simulink model "Design_of_an_Energy_Efficient_Hybrid_Electric_Vehicle"  (R2023a)
settings: Solver=FixedStepDiscrete  StartTime=0  StopTime=110  RelTol=1e-3  EnableMultiTasking=on
PreLoadFcn:
  | power_motordrive_IPMSM_FOC_data
InitFcn:
  | power_motordrive_IPMSM_FOC_data
  | Cdc  = 0.001;      % DC-link capacitor  [F]
  | AH0  = 280;        % Initial battery charge [hr*A]
  | Tmax=410;
  | 
  | %% Vehicle Parameters for Vehicle Dynamics 2
  | vehicle_mass = 2111;
  | wheel_radius = 0.228;
  | area =2.22;
  | drag_coefficient = 0.23;
  | air_density = 1.204;
  | gravity = 9.81;
  | rolling_res_ratio = 0.02;
  | 
  | % Differential drive parameters
  | gear_ratio = 5;
  | i_t   = gear_ratio ;
  | Rw=wheel_radius;
  | 
  | 
  | %% Sliding Mode Observer
  | pmsm.N_max=wmax;
  | pmsm.p=p
  | pmsm.Ld=Ld;
  | pmsm.Lq=Lq;
  | pmsm.Rs=Rs;
  | PU_System.V_base=(Vdc_nom/sqrt(3));
  | PU_System.I_base=lambda/(Lq-Ld);
  | max_torque=400
  | force_max_pedal=500
  | braking_torque_to_pedal_force_ratio=-4
undefined symbols (not defined in the file): BlkSampleTime, CurrentObserverGain, dataType, DiscIntNeverNeededParam, Fsw, gcbh, Ki_Ireg, Ki_wreg, Kp_Ireg, Kp_wreg, L_smo_gain, lambda, Ld, Limit_Ireg, Limit_wreg, Lq, MaxApplicationSpeed, MaxStatorCurrent, MaxStatorVoltage, NumBits1, NumBits2, p, Pmsm, PolePairs, QPLL, rpm_data, Sensorless, sigbuilder_block, SlidingLimit, Slope1, Slope2, sps_rtmsupport, StatorInductance, StatorResistance, Tmax_data, Tnom, Ts, Vdc_nom, wmax
libraries: fl_lib x27, nesl_utility x24, simulink x23, mcbcontrolslib x15, fl_ps_legacy_lib x9, spsStairGeneratorLib x7, sdl_lib x6, ee_lib x4, mcbpositiondecoderlib x4, BoomBox x3, tiiqmathlib x2, autolibshared x2
(part 4 of 4)

== system Design_of_an_Energy_Efficient_Hybrid_Electric_Vehicle/FOC/Speed Regulator1/Calculate position and speed/Sliding Mode Observer/EEMF Model/angleCompensation ==
  A : Inport
  B : Inport  Port=2
  C : Inport  Port=3
  D : Inport  Port=4
  Bias : Bias  Bias=single(2*pi)  SaturateOnIntegerOverflow=off
  Data Type Duplicate : DataTypeDuplicate  NumInputPorts=6
  Data Type Propagation : simulink/Signal Attributes/Data Type Propagation  PropDataType=fixdt(1, 16)  IfRefDouble=double  IfRefSingle=single  IsSigned=IsSigned1 or IsSigned2  NumBitsBase=max([NumBits1 NumBits2])  NumBitsMult=1  NumBitsAdd=0  NumBitsAllowFinal=1:128  PropScalingMode=Obtain via best precision  PropScaling=2^-10  ValuesUsedBestPrec=[2*pi -2*pi]  SlopeBase=min([Slope1 Slope2])  SlopeMult=1  SlopeAdd=0  BiasBase=Bias1  BiasMult=1  BiasAdd=0
  Data Type Conversion : DataTypeConversion  SaturateOnIntegerOverflow=off  RndMeth=Floor
  Product{,1..3} (4 alike) : Product  OutDataTypeStr=Inherit: Inherit via back propagation
  Scope : Scope
  Sum1 : Sum  Inputs=|++  OutDataTypeStr=Inherit: Same as first input
  Sum2 : Sum  Inputs=|+-  OutDataTypeStr=Inherit: Same as first input
  Switch : Switch  Criteria=u2 > Threshold  SaturateOnIntegerOverflow=off  InputSameDT=off
  atan1 : mcbcontrolslib/atan2  outputUnit=Radians
  Theta : Outport
  wires:
  Data Type Conversion/1 -> Bias/1, Data Type Propagation/3, Switch/2, Switch/1
  Sum1/1 -> atan1/1
  Sum2/1 -> atan1/2
  B/1 -> Product1/1, Product2/1
  atan1/1 -> Scope/1, Data Type Conversion/1, Data Type Propagation/2, Data Type Propagation/1
  D/1 -> Product1/2, Product/2, Data Type Duplicate/6
  C/1 -> Product3/2, Data Type Duplicate/1, Product2/2
  A/1 -> Product3/1, Product/1
  Product2/1 -> Sum1/2, Data Type Duplicate/4
  Switch/1 -> Theta/1
  Bias/1 -> Switch/3
  Product3/1 -> Sum2/2, Data Type Duplicate/2
  Product/1 -> Sum1/1, Data Type Duplicate/5
  Product1/1 -> Sum2/1, Data Type Duplicate/3

== system Design_of_an_Energy_Efficient_Hybrid_Electric_Vehicle/FOC/Speed Regulator1/Calculate position and speed/Sliding Mode Observer/Sliding Mode Observer/Direction_Latch ==
  SigmaAlpha : Inport
  SigmaBeta : Inport  Port=2
  Compare To Zero : simulink/Logic and Bit Operations/Compare To Zero  relop=>  OutDataTypeStr=boolean
  Compare To Zero1 : simulink/Logic and Bit Operations/Compare To Zero  relop=>  OutDataTypeStr=boolean
  Dir_Sense : Subsystem  TreatAsAtomicUnit=on
  If : If
  Merge : Merge
  Merge1 : Merge
  Subsystem2 : Subsystem
  Subsystem3 : Subsystem
  A : Outport
  B : Outport  Port=2
  wires:
  Dir_Sense/1(Sign) -> If/1
  Compare To Zero/1 -> Dir_Sense/1(A), Dir_Sense/Trigger
  Compare To Zero1/1 -> Dir_Sense/2(B)
  Merge/1 -> A/1
  Merge1/1 -> B/1
  Subsystem2/2(Out2) -> Merge1/1
  Subsystem3/1(Out2) -> Merge1/2
  If/2 -> Subsystem3/Action
  Subsystem3/2(Out1) -> Merge/2
  Subsystem2/1(Out1) -> Merge/1
  If/1 -> Subsystem2/Action
  SigmaBeta/1 -> Compare To Zero1/1, Subsystem2/2(SigmaBeta), Subsystem3/1(SigmaBeta)
  SigmaAlpha/1 -> Subsystem3/2(SigmaAlpha), Subsystem2/1(SigmaAlpha), Compare To Zero/1

== system Design_of_an_Energy_Efficient_Hybrid_Electric_Vehicle/FOC/Speed Regulator1/Calculate position and speed/Sliding Mode Observer/Sliding Mode Observer/Subsystem ==
  note: Back Emf computation
  note: Ialpha Estimation
  Valpha : Inport
  Ialpha : Inport  Port=2
  Reset : Inport  Port=3
  Data Type Duplicate : DataTypeDuplicate
  Data Type Duplicate1 : DataTypeDuplicate  NumInputPorts=3
  Data Type Propagation : simulink/Signal Attributes/Data Type Propagation  PropDataType=fixdt(1, 16)  IfRefDouble=double  IfRefSingle=single  IsSigned=IsSigned1 or IsSigned2  NumBitsBase=max([NumBits1 NumBits2])  NumBitsMult=1  NumBitsAdd=0  NumBitsAllowFinal=1:128  PropScalingMode=Obtain via best precision  PropScaling=2^-10  ValuesUsedBestPrec=[SlidingLimit*CurrentObserverGain -SlidingLimit*CurrentObserverGain]  SlopeBase=min([Slope1 Slope2])  SlopeMult=1  SlopeAdd=0  BiasBase=Bias1  BiasMult=1  BiasAdd=0
  Delay : Delay  DelayLength=1  ExternalReset=Level
      settings: InputPortMap=u0,r5
  Delay1 : Delay  DelayLength=1  ExternalReset=Level
      settings: InputPortMap=u0,r5
  Foc_gain : Gain  Gain=single(CurrentObserverGain)  OutDataTypeStr=Inherit: Inherit via back propagation
  Gain : Gain  Gain=single((1/StatorResistance)*(1-exp(-StatorResistance*BlkSampleTime(1)/StatorInductance))*(MaxStatorVoltage/sqrt(3))/MaxStatorCurrent)  OutDataTypeStr=Inherit: Same as input
  Gain1 : Gain  Gain=single(exp(-StatorResistance*BlkSampleTime(1)/StatorInductance))  OutDataTypeStr=Inherit: Same as input
  Gain2 : Gain  Gain=single(2*pi*MaxApplicationSpeed*PolePairs*(1/60)*2*BlkSampleTime(1))  OutDataTypeStr=Inherit: Same as input
  Saturation : Saturate  UpperLimit=SlidingLimit  LowerLimit=-1*SlidingLimit
  Sum : Sum  Inputs=|-+  OutDataTypeStr=Inherit: Same as first input
  Sum1 : Sum  Inputs=+-|  OutDataTypeStr=Inherit: Same as first input
  Sum2 : Sum  OutDataTypeStr=Inherit: Same as first input
  Sum3 : Sum  Inputs=-+|  OutDataTypeStr=Inherit: Same as first input
  Sum4 : Sum  Inputs=++|  OutDataTypeStr=Inherit: Inherit via back propagation
  SigmaAlpha : Outport  VectorParamsAs1DForOutWhenUnconnected=off
  wires:
  Reset/1 -> Delay/2, Delay1/2
  Sum/1 -> Saturation/1, Data Type Propagation/2, Data Type Propagation/1
  Ialpha/1 -> Sum/1, Data Type Duplicate1/1
  Valpha/1 -> Sum1/1, Data Type Duplicate/1
  Gain1/1 -> Sum2/2
  Gain/1 -> Sum2/1, Data Type Duplicate1/3
  Sum1/1 -> Gain/1
  Delay/1 -> Gain1/1
  Sum4/1 -> Delay1/1, Data Type Duplicate/2
  Sum2/1 -> Delay/1, Sum/2, Data Type Duplicate1/2
  Delay1/1 -> Sum1/2, Sum3/1, SigmaAlpha/1, Sum4/1
  Saturation/1 -> Foc_gain/1
  Foc_gain/1 -> Data Type Propagation/3, Sum3/2
  Sum3/1 -> Gain2/1
  Gain2/1 -> Sum4/2

== system Design_of_an_Energy_Efficient_Hybrid_Electric_Vehicle/FOC/Speed Regulator1/Calculate position and speed/Sliding Mode Observer/Sliding Mode Observer/Subsystem1 ==
  note: Back Emf computation
  note: Ibeta Estimation
  Vbeta : Inport
  Ibetaa : Inport  Port=2
  Reset : Inport  Port=3
  Data Type Duplicate : DataTypeDuplicate
  Data Type Duplicate1 : DataTypeDuplicate  NumInputPorts=3
  Data Type Propagation : simulink/Signal Attributes/Data Type Propagation  PropDataType=fixdt(1, 16)  IfRefDouble=double  IfRefSingle=single  IsSigned=IsSigned1 or IsSigned2  NumBitsBase=max([NumBits1 NumBits2])  NumBitsMult=1  NumBitsAdd=0  NumBitsAllowFinal=1:128  PropScalingMode=Obtain via best precision  PropScaling=2^-10  ValuesUsedBestPrec=[SlidingLimit*CurrentObserverGain -SlidingLimit*CurrentObserverGain]  SlopeBase=min([Slope1 Slope2])  SlopeMult=1  SlopeAdd=0  BiasBase=Bias1  BiasMult=1  BiasAdd=0
  Delay : Delay  DelayLength=1  ExternalReset=Level
      settings: InputPortMap=u0,r5
  Delay1 : Delay  DelayLength=1  ExternalReset=Level
      settings: InputPortMap=u0,r5
  Foc_gain : Gain  Gain=single(CurrentObserverGain)  OutDataTypeStr=Inherit: Inherit via back propagation
  Gain : Gain  Gain=single((1/StatorResistance)*(1-exp(-StatorResistance*BlkSampleTime(1)/StatorInductance))*(MaxStatorVoltage/sqrt(3))/MaxStatorCurrent)  OutDataTypeStr=Inherit: Same as input
  Gain1 : Gain  Gain=single(exp(-StatorResistance*BlkSampleTime(1)/StatorInductance))  OutDataTypeStr=Inherit: Same as input
  Gain2 : Gain  Gain=single(2*pi*MaxApplicationSpeed*PolePairs*(1/60)*2*BlkSampleTime(1))  OutDataTypeStr=Inherit: Same as input
  Saturation : Saturate  UpperLimit=SlidingLimit  LowerLimit=-1*SlidingLimit
  Sum : Sum  Inputs=|-+  OutDataTypeStr=Inherit: Same as first input
  Sum1 : Sum  Inputs=+-|  OutDataTypeStr=Inherit: Same as first input
  Sum2 : Sum  OutDataTypeStr=Inherit: Same as first input
  Sum3 : Sum  Inputs=-+|  OutDataTypeStr=Inherit: Same as first input
  Sum4 : Sum  Inputs=++|  OutDataTypeStr=Inherit: Inherit via back propagation
  SigmaBeta : Outport  VectorParamsAs1DForOutWhenUnconnected=off
  wires:
  Reset/1 -> Delay1/2, Delay/2
  Sum/1 -> Saturation/1, Data Type Propagation/2, Data Type Propagation/1
  Ibetaa/1 -> Sum/1, Data Type Duplicate1/1
  Vbeta/1 -> Sum1/1, Data Type Duplicate/1
  Gain1/1 -> Sum2/2
  Saturation/1 -> Foc_gain/1
  Gain/1 -> Sum2/1, Data Type Duplicate1/3
  Sum1/1 -> Gain/1
  Foc_gain/1 -> Sum3/2, Data Type Propagation/3
  Delay/1 -> Gain1/1
  Sum4/1 -> Delay1/1, Data Type Duplicate/2
  Sum2/1 -> Delay/1, Sum/2, Data Type Duplicate1/2
  Delay1/1 -> Sum1/2, Sum3/1, SigmaBeta/1, Sum4/1
  Sum3/1 -> Gain2/1
  Gain2/1 -> Sum4/2

== system Design_of_an_Energy_Efficient_Hybrid_Electric_Vehicle/FOC/Speed Regulator1/Calculate position and speed/Sliding Mode Observer/Sliding Mode Observer/angleCompensation ==
  A : Inport
  B : Inport  Port=2
  C : Inport  Port=3
  D : Inport  Port=4
  Bias : Bias  Bias=single(2*pi)  SaturateOnIntegerOverflow=off
  Data Type Duplicate : DataTypeDuplicate  NumInputPorts=6
  Data Type Propagation : simulink/Signal Attributes/Data Type Propagation  PropDataType=fixdt(1, 16)  IfRefDouble=double  IfRefSingle=single  IsSigned=IsSigned1 or IsSigned2  NumBitsBase=max([NumBits1 NumBits2])  NumBitsMult=1  NumBitsAdd=0  NumBitsAllowFinal=1:128  PropScalingMode=Obtain via best precision  PropScaling=2^-10  ValuesUsedBestPrec=[2*pi -2*pi]  SlopeBase=min([Slope1 Slope2])  SlopeMult=1  SlopeAdd=0  BiasBase=Bias1  BiasMult=1  BiasAdd=0
  Data Type Conversion : DataTypeConversion  SaturateOnIntegerOverflow=off  RndMeth=Floor
  Product{,1..3} (4 alike) : Product  OutDataTypeStr=Inherit: Inherit via back propagation
  Sum1 : Sum  Inputs=|++  OutDataTypeStr=Inherit: Same as first input
  Sum2 : Sum  Inputs=|+-  OutDataTypeStr=Inherit: Same as first input
  Switch : Switch  Criteria=u2 > Threshold  SaturateOnIntegerOverflow=off  InputSameDT=off
  atan1 : mcbcontrolslib/atan2  outputUnit=Radians
  Theta : Outport
  wires:
  Data Type Conversion/1 -> Bias/1, Data Type Propagation/3, Switch/2, Switch/1
  Sum1/1 -> atan1/1
  Sum2/1 -> atan1/2
  B/1 -> Product1/1, Product2/1
  atan1/1 -> Data Type Conversion/1, Data Type Propagation/2, Data Type Propagation/1
  D/1 -> Product1/2, Product/2, Data Type Duplicate/6
  C/1 -> Product3/2, Data Type Duplicate/1, Product2/2
  A/1 -> Product3/1, Product/1
  Product2/1 -> Sum1/2, Data Type Duplicate/4
  Switch/1 -> Theta/1
  Bias/1 -> Switch/3
  Product3/1 -> Sum2/2, Data Type Duplicate/2
  Product/1 -> Sum1/1, Data Type Duplicate/5
  Product1/1 -> Sum2/1, Data Type Duplicate/3

== system Design_of_an_Energy_Efficient_Hybrid_Electric_Vehicle/FOC/Speed Regulator1/Calculate position and speed/Sliding Mode Observer/Subsystem/Alpha_loop_current_est ==
  Valpha : Inport
  Ialpha : Inport  Port=2
  Reset1 : Inport  Port=3
  Add : Sum  Inputs=-+
  Eq12_alpha_loop : Subsystem
  Gain3 : Gain  Gain=L_smo_gain  OutDataTypeStr=Inherit: Same as input
  Saturation : Saturate  UpperLimit=SlidingLimit  LowerLimit=-1*SlidingLimit  OutDataTypeStr=single
  Zalpha[k+1] : Outport  VectorParamsAs1DForOutWhenUnconnected=off
  wires:
  Valpha/1 -> Eq12_alpha_loop/2(Valpha*)
  Eq12_alpha_loop/1(Ialpha_est) -> Add/2
  Ialpha/1 -> Add/1
  Add/1 -> Saturation/1
  Saturation/1 -> Gain3/1, Zalpha[k+1]/1
  Gain3/1 -> Eq12_alpha_loop/1(L*Zalpha[k+1])
  Reset1/1 -> Eq12_alpha_loop/3(Reset)

== system Design_of_an_Energy_Efficient_Hybrid_Electric_Vehicle/FOC/Speed Regulator1/Calculate position and speed/Sliding Mode Observer/Subsystem/Beta_loop_current_est ==
  Vbeta : Inport
  Ibeta : Inport  Port=2
  Reset1 : Inport  Port=3
  Add : Sum  Inputs=-+
  Eq12_beta_loop : Subsystem
  Gain3 : Gain  Gain=L_smo_gain  OutDataTypeStr=Inherit: Same as input
  Saturation : Saturate  UpperLimit=SlidingLimit  LowerLimit=-1*SlidingLimit  OutDataTypeStr=single
  Zbeta[k+1] : Outport  VectorParamsAs1DForOutWhenUnconnected=off
  wires:
  Vbeta/1 -> Eq12_beta_loop/2(Vbeta*)
  Eq12_beta_loop/1(Ibeta_est) -> Add/2
  Ibeta/1 -> Add/1
  Add/1 -> Saturation/1
  Saturation/1 -> Gain3/1, Zbeta[k+1]/1
  Gain3/1 -> Eq12_beta_loop/1(L*Zbeta[k+1])
  Reset1/1 -> Eq12_beta_loop/3(Reset)

== system Design_of_an_Energy_Efficient_Hybrid_Electric_Vehicle/FOC/Speed Regulator1/Calculate position and speed/Sliding Mode Observer/Subsystem/QPLL ==
  Zalpha[k+1] : Inport
  Zbeta[k+1] : Inport  Port=2
  Add : Sum
  Add1 : Sum  Inputs=--
  Demux : Demux  Outputs=2
  Divide : Product  Inputs=/*  OutDataTypeStr=double
  Gain2 : Gain  Gain=single(60/((2*pi)*pmsm.N_base*pmsm.p))
  IIR Filter2 : mcbcontrolslib/IIR Filter  VariantControl=Low Pass Filter  VariantSelect=Low-pass  Filter_constant=single(Ts*pmsm.N_max*pmsm.p/120)  advancedSettings=off  Ts=50e-6  cutOff_freq=1
  Math Function : Math  Operator=square
  Math Function1 : Math  Operator=square
  Mux : Mux  Inputs=2
  PI Controller : slpidlib/PID Controller  Controller=PI  Form=Parallel  TimeDomain=Discrete-time  UseExternalTs=off  SampleTime=-1  IntegratorMethod=Forward Euler  FilterMethod=Forward Euler  ControllerParametersSource=internal  P=90  I=300  D=0  UseFilter=on  N=100  TunerSelectOption=Transfer Function Based (PID Tuner App)  InitialConditionSource=internal  InitialConditionForIntegrator=0  InitialConditionForFilter=0  DifferentiatorICPrevScaledInput=0  ExternalReset=none  TrackingMode=off  Kt=1  LimitOutput=off  SatLimitsSource=internal  UpperSaturationLimit=inf  LowerSaturationLimit=0  LinearizeAsGain=off  AntiWindupMode=none  Kb=1  POutMin=[]  POutMax=[]  IOutMin=[]  IOutMax=[]  DOutMin=[]  DOutMax=[]  NOutMin=[]  NOutMax=[]  SumOutMin=[]  SumOutMax=[]  SaturationOutMin=[]  SaturationOutMax=[]  PParamMin=[]  PParamMax=[]  IParamMin=[]  IParamMax=[]  DParamMin=[]  DParamMax=[]  NParamMin=[]  NParamMax=[]  KbParamMin=[]  KbParamMax=[]  KtParamMin=[]  KtParamMax=[]  KbOutMin=[]  KbOutMax=[]  KtOutMin=[]  KtOutMax=[]  IntegratorOutMin=[]  IntegratorOutMax=[]  FilterOutMin=[]  FilterOutMax=[]  SumI1OutMin=[]  SumI1OutMax=[]  SumI2OutMin=[]  SumI2OutMax=[]  SumI3OutMin=[]  SumI3OutMax=[]  SumI4OutMin=[]  SumI4OutMax=[]  SumDOutMin=[]  SumDOutMax=[]  DifferentiatorOutMin=[]  DifferentiatorOutMax=[]  FilterDiffOutCoefMin=[]  FilterDiffOutCoefMax=[]  ReciprocalOutMin=[]  ReciprocalOutMax=[]  SumDenOutMin=[]  SumDenOutMax=[]  SumNumOutMin=[]  SumNumOutMax=[]  DivideOutMin=[]  DivideOutMax=[]  UdiffTsProdOutMin=[]  UdiffTsProdOutMax=[]  NTsProdOutMin=[]  NTsProdOutMax=[]  UintegralTsProdOutMin=[]  UintegralTsProdOutMax=[]  UngainTsProdOutMin=[]  UngainTsProdOutMax=[]  IntegratorContinuousStateAttributes=''  IntegratorStateMustResolveToSignalObject=off  IntegratorRTWStateStorageClass=Auto  FilterContinuousStateAttributes=''  FilterStateMustResolveToSignalObject=off  FilterRTWStateStorageClass=Auto  ParallelPVariant=InternalParameters  IdealPVariant=Disabled  IVariant=InternalParameters  DVariant=Disabled  IntegratorVariant=Discrete  SatVariant=Disabled  AWVariant=Passthrough  PCopyVariant=Disabled  TRVariant=Disabled  FdbkBlocksVariant=Forward  IdealPFdbkVariant=Disabled  SatFdbkVariant=Disabled  DerivativeFilterVariant=Disabled  NVariant=Disabled  NCopyVariant=Disabled_SignalSpec  FilterICVariant=Disabled  IntegratorICVariant=InternalICs  ExternalResetVariant=Disabled  TRSumVariant=Passthrough  SumFdbkVariant=Disabled  SumVariant=Sum_PI  TsampFilterVariant=InternalTs  TsampNgainVariant=Passthrough  TsampIntegralVariant=Passthrough  ExternalSaturationOutDataTypeStr=Inherit: Same as second input
  Product : Product  OutDataTypeStr=Inherit: Inherit via back propagation
  Product1 : Product  OutDataTypeStr=Inherit: Inherit via back propagation
  Scope{1..3,5,7} (5 alike) : Scope  NumInputPorts=2
  Sqrt : Sqrt
  Trigonometric Function : Trigonometry  Operator=cos  OutputSignalType=real
  Trigonometric Function1 : Trigonometry  OutputSignalType=real
  Wrap state discrete Integrator : Subsystem  AncestorBlock=|
      | eeAsmScalarControl/Induction Machine
      | Scalar Control/Wrap state
      | discrete Integrator
      settings: LibrarySourceBlock=|
      | eeAsmScalarControl/Induction Machine
      | Scalar Control/Wrap state
      | discrete Integrator
  y : Outport
  wires:
  Math Function/1 -> Add/1
  Math Function1/1 -> Add/2
  Add/1 -> Sqrt/1
  Demux/1 -> Math Function/1, Product/2, Scope2/1
  Demux/2 -> Math Function1/1, Product1/1, Scope2/2
  Product/1 -> Add1/1
  Product1/1 -> Add1/2
  Divide/1 -> Scope7/2, PI Controller/1
  Zalpha[k+1]/1 -> Mux/2
  Zbeta[k+1]/1 -> Mux/1
  Sqrt/1 -> Divide/1, Scope3/1
  Add1/1 -> Divide/2, Scope7/1
  Trigonometric Function/1 -> Product1/2
  Trigonometric Function1/1 -> Product/1
  Wrap state discrete Integrator/1(y) -> Trigonometric Function/1, Trigonometric Function1/1, Scope1/1, y/1
  Gain2/1 -> Scope1/2
  Mux/1 -> Demux/1
  PI Controller/1 -> IIR Filter2/1, Wrap state discrete Integrator/1(u)
  IIR Filter2/1 -> Gain2/1

== system Design_of_an_Energy_Efficient_Hybrid_Electric_Vehicle/FOC/Speed Regulator1/Calculate position and speed/Sliding Mode Observer (SMO)/Debounce/Speed IIR filter ==
  Speed : Inport
  Add : Sum  Inputs=+-
  Add1 : Sum
  Constant1 : Constant  OutDataTypeStr=fixdt(1,32,17)
  Constant2 : Constant  Value=.01  OutDataTypeStr=fixdt(1,32,17)
  Product : Product  OutDataTypeStr=Inherit: Same as first input
  Product1 : Product  OutDataTypeStr=Inherit: Same as first input
  Unit Delay : UnitDelay  SampleTime=-1  HasFrameUpgradeWarning=on
  Filtered speed : Outport  VectorParamsAs1DForOutWhenUnconnected=off
  wires:
  Speed/1 -> Product/1
  Add1/1 -> Unit Delay/1, Filtered speed/1
  Constant1/1 -> Add/1
  Constant2/1 -> Product/2, Add/2
  Product/1 -> Add1/1
  Add/1 -> Product1/1
  Unit Delay/1 -> Product1/2
  Product1/1 -> Add1/2

== system Design_of_an_Energy_Efficient_Hybrid_Electric_Vehicle/FOC/Speed Regulator1/Calculate position and speed/Sliding Mode Observer/EEMF Model/Direction_Latch/Dir_Sense ==
  A : Inport
  B : Inport  Port=2
  Trigger : TriggerPort  VariantControl=Variant
  Constant : Constant  Value=-1
  Constant1 : Constant
  Logical Operator : Logic  AllPortsSameDT=off  OutDataTypeStr=boolean
  Switch : Switch  Criteria=u2 ~= 0  OutDataTypeStr=int16  SaturateOnIntegerOverflow=off  InputSameDT=off
  Sign : Outport  InitialOutput=0  VectorParamsAs1DForOutWhenUnconnected=off
  wires:
  Switch/1 -> Sign/1
  Constant1/1 -> Switch/3
  Constant/1 -> Switch/1
  Logical Operator/1 -> Switch/2
  B/1 -> Logical Operator/2
  A/1 -> Logical Operator/1

== system Design_of_an_Energy_Efficient_Hybrid_Electric_Vehicle/FOC/Speed Regulator1/Calculate position and speed/Sliding Mode Observer/EEMF Model/Direction_Latch/Subsystem2 ==
  SigmaAlpha : Inport
  SigmaBeta : Inport  Port=2
  Action Port : ActionPort  ActionPortLabel=if(u1 > 0)
  Unary Minus : UnaryMinus
  Out1 : Outport
  Out2 : Outport  Port=2
  wires:
  Unary Minus/1 -> Out1/1
  SigmaBeta/1 -> Out2/1
  SigmaAlpha/1 -> Unary Minus/1

== system Design_of_an_Energy_Efficient_Hybrid_Electric_Vehicle/FOC/Speed Regulator1/Calculate position and speed/Sliding Mode Observer/EEMF Model/Direction_Latch/Subsystem3 ==
  SigmaBeta : Inport
  SigmaAlpha : Inport  Port=2
  Action Port : ActionPort  ActionPortLabel=else
  Unary Minus : UnaryMinus
  Out2 : Outport
  Out1 : Outport  Port=2
  wires:
  Unary Minus/1 -> Out2/1
  SigmaAlpha/1 -> Out1/1
  SigmaBeta/1 -> Unary Minus/1

== system Design_of_an_Energy_Efficient_Hybrid_Electric_Vehicle/FOC/Speed Regulator1/Calculate position and speed/Sliding Mode Observer/EEMF Model/Sliding Mode Observer/2nd order LPF ==
  In : Inport
  reset : Inport  Port=2
  Compute filter constant : Subsystem
  LPF1 : Subsystem  mask(Basic IIR LPF filter){}
      mask help:
      | The output is computed as:
      | y[k] = G * y[k-1] + (1-G) * u[k]
  LPF2 : Subsystem  mask(Basic IIR LPF filter){}
      mask help:
      | The output is computed as:
      | y[k] = G * y[k-1] + (1-G) * u[k]
  Out : Outport
  wires:
  reset/1 -> LPF2/2(rst), LPF1/2(rst)
  In/1 -> LPF1/1(In)
  Compute filter constant/1(G) -> LPF1/3(G), LPF2/3(G)
  LPF1/1(Out) -> LPF2/1(In)
  LPF2/1(Out) -> Out/1

== system Design_of_an_Energy_Efficient_Hybrid_Electric_Vehicle/FOC/Speed Regulator1/Calculate position and speed/Sliding Mode Observer/EEMF Model/Sliding Mode Observer/Back EMF estimation (SMO) ==
  Is_αβ : Inport
  Vs_αβ : Inport  Port=2
  Delay : Delay  DelayLength=1  InitialCondition=0
  Gain1 : Gain  Gain=Rs/Ls
  Gain2 : Gain  Gain=1/Ls
  Gain3 : Gain  Gain=Ks
  Gain4 : Gain  Gain=1/Ls
  Sigmoid : Subsystem
      mask Display: plot(linspace(-1,1,100),(2./(1+exp(-10*linspace(-1,1,100))))-1)
  Sum : Sum  Inputs=|++
  Sum1 : Sum  Inputs=|+-
  Sum2 : Sum  Inputs=|+-
  Sum3 : Sum  Inputs=|-+
  Weighted sample time : SampleTimeMath  TsampMathOp=*  weightValue=1
  Weighted sample time1 : SampleTimeMath  TsampMathOp=*  weightValue=1
  Weighted sample time2 : SampleTimeMath  TsampMathOp=*  weightValue=1
  e_αβ : Outport
  wires:
  Sum/1 -> Sum1/1
  Sum1/1 -> Delay/1
  Sum3/1 -> Sum/1
  Gain4/1 -> Sum/2
  Is_αβ/1 -> Sum2/2
  Vs_αβ/1 -> Weighted sample time1/1
  Delay/1 -> Weighted sample time2/1, Sum3/2, Sum2/1
  Gain3/1 -> e_αβ/1, Weighted sample time/1
  Sum2/1 -> Sigmoid/1(u)
  Sigmoid/1(y) -> Gain3/1
  Weighted sample time/1 -> Gain2/1
  Gain2/1 -> Sum1/2
  Weighted sample time1/1 -> Gain4/1
  Weighted sample time2/1 -> Gain1/1
  Gain1/1 -> Sum3/1

== system Design_of_an_Energy_Efficient_Hybrid_Electric_Vehicle/FOC/Speed Regulator1/Calculate position and speed/Sliding Mode Observer/EEMF Model/Sliding Mode Observer/Speed//position estimation Arctan method ==
  e_αβ : Inport
  reset : Inport  Port=2
  Atan : Trigonometry  Operator=atan2
  Demux : Demux  Outputs=2
  Gain : Gain  Gain=-1
  Rotor mechanical speed : Subsystem  mask{fc=1e3}
      mask prompts: fc "Filter cutoff frequency [Hz]"
      mask help:
      | The rotor speed is obtained by differentiation of the measured angle. The "function block" removes angle discontinuities.
      |
      | The derivative is then filtered to reduce the noise introduced by the numerical differentiation.
      |
      | Additional details can be found in "PN104: Using the angle decoder modules" on the imperix knowledge base (kb.imperix.com).
  Scope1 : Scope
  Scope2 : Scope
  Scope3 : Scope
  ωs : Outport
  θs : Outport  Port=2
  wires:
  Demux/1 -> Atan/1
  Demux/2 -> Atan/2
  e_αβ/1 -> Demux/1
  Atan/1 -> Scope2/1, Gain/1
  Gain/1 -> Rotor mechanical speed/1(angle), θs/1
  Rotor mechanical speed/1(speed) -> Scope3/1, ωs/1
  reset/1 -> Scope1/1, Rotor mechanical speed/2(reset)

== system Design_of_an_Energy_Efficient_Hybrid_Electric_Vehicle/FOC/Speed Regulator1/Calculate position and speed/Sliding Mode Observer/EEMF Model/Sliding Mode Observer/Speed//position estimation Q-PLL method ==
  V_αβ : Inport
  ωc : Inport  Port=2
  Kp : Inport  Port=3
  Ki : Inport  Port=4
  reset : Inport  Port=5
  Constant : Constant  Value=[0 0]  OutDataTypeStr=single
  Demux : Demux  Outputs=2
  PI : Subsystem
  Product : Product
  Product1 : Product
  Sum : Sum  Inputs=|++
  Sum1 : Sum  Inputs=-|+
  Switch : Switch  Criteria=u2 > Threshold  SaturateOnIntegerOverflow=off  InputSameDT=off
  Trigonometric Function : Trigonometry  OutputSignalType=real
  Trigonometric Function1 : Trigonometry  Operator=cos  OutputSignalType=real
  Wrapping integrator : Subsystem
      mask help: The integrator uses the Forward Euler method and wraps its state between 0 and 2*pi.
  ωs : Outport
  θs : Outport  Port=2
  wires:
  reset/1 -> PI/4(Reset), Switch/2
  PI/1(u) -> Sum/1
  Switch/1 -> Demux/1
  V_αβ/1 -> Switch/3
  Constant/1 -> Switch/1
  Trigonometric Function/1 -> Product1/1
  Trigonometric Function1/1 -> Product/2
  Sum1/1 -> PI/1(e)
  Demux/1 -> Product1/2
  Demux/2 -> Product/1
  Wrapping integrator/1(out) -> θs/1, Trigonometric Function1/1, Trigonometric Function/1
  Sum/1 -> Wrapping integrator/1(in), ωs/1
  ωc/1 -> Sum/2
  Kp/1 -> PI/2(Kp)
  Ki/1 -> PI/3(Ki)
  Product1/1 -> Sum1/1
  Product/1 -> Sum1/2

== system Design_of_an_Energy_Efficient_Hybrid_Electric_Vehicle/FOC/Speed Regulator1/Calculate position and speed/Sliding Mode Observer/EEMF Model/Sliding Mode Observer/compensate LPF phase 1 ==
  ωs : Inport
  θ_in : Inport  Port=2
  Add : Sum
  Atan : Trigonometry  Operator=atan2
  Constant1 : Constant  Value=2*pi*fc  OutDataTypeStr=single
  Filter order : Gain  Gain=2
  θ_out : Outport
  wires:
  Constant1/1 -> Atan/2
  ωs/1 -> Atan/1
  Add/1 -> θ_out/1
  Atan/1 -> Filter order/1
  θ_in/1 -> Add/1
  Filter order/1 -> Add/2

== system Design_of_an_Energy_Efficient_Hybrid_Electric_Vehicle/FOC/Speed Regulator1/Calculate position and speed/Sliding Mode Observer/EEMF Model/Sliding Mode Observer/compensate LPF phase 2 ==
  ωs : Inport
  θ_in : Inport  Port=2
  Add : Sum
  Atan : Trigonometry  Operator=atan2
  Constant1 : Constant  Value=2*pi*fc  OutDataTypeStr=single
  Filter order : Gain  Gain=2
  θ_out : Outport
  wires:
  Filter order/1 -> Add/2
  θ_in/1 -> Add/1
  Atan/1 -> Filter order/1
  Add/1 -> θ_out/1
  ωs/1 -> Atan/1
  Constant1/1 -> Atan/2

== system Design_of_an_Energy_Efficient_Hybrid_Electric_Vehicle/FOC/Speed Regulator1/Calculate position and speed/Sliding Mode Observer/EEMF Model/Sliding Mode Observer/compensate PLL phase ==
  θ_in : Inport
  ωc : Inport  Port=2
  Gain : Gain  Gain=pi/2
  Sign : Signum
  Sum : Sum  Inputs=|+-
  θ_out : Outport
  wires:
  θ_in/1 -> Sum/1
  Sum/1 -> θ_out/1
  Sign/1 -> Gain/1
  ωc/1 -> Sign/1
  Gain/1 -> Sum/2

== system Design_of_an_Energy_Efficient_Hybrid_Electric_Vehicle/FOC/Speed Regulator1/Calculate position and speed/Sliding Mode Observer/EEMF Model/Subsystem/shi_1 ==
  In1 : Inport
  Gain : Gain  Gain=-1
  Gain8 : Gain  Gain=single((pmsm.Ld-pmsm.Lq))
  Gain9 : Gain
  Shi1 : Gain  Gain=single((1/pmsm.Rs)*(1-exp(-pmsm.Rs*Ts/pmsm.Ld))*(PU_System.V_base/sqrt(3))/PU_System.I_base)  OutDataTypeStr=Inherit: Same as input
  Out1 : Outport
  wires:
  Gain8/1 -> Out1/1
  Gain9/1 -> Shi1/1
  In1/1 -> Gain/1
  Gain/1 -> Gain9/1
  Shi1/1 -> Gain8/1

== system Design_of_an_Energy_Efficient_Hybrid_Electric_Vehicle/FOC/Speed Regulator1/Calculate position and speed/Sliding Mode Observer/EEMF Model/Subsystem1/shi_1 ==
  In1 : Inport
  Gain : Gain
  Gain8 : Gain  Gain=single((pmsm.Ld-pmsm.Lq))
  Gain9 : Gain
  Shi : Gain  Gain=single((1/pmsm.Rs)*(1-exp(-pmsm.Rs*Ts/pmsm.Ld))*(PU_System.V_base/sqrt(3))/PU_System.I_base)  OutDataTypeStr=Inherit: Same as input
  Out1 : Outport
  wires:
  Gain8/1 -> Out1/1
  Gain9/1 -> Shi/1
  In1/1 -> Gain/1
  Gain/1 -> Gain9/1
  Shi/1 -> Gain8/1

== system Design_of_an_Energy_Efficient_Hybrid_Electric_Vehicle/FOC/Speed Regulator1/Calculate position and speed/Sliding Mode Observer/Sliding Mode Observer/Direction_Latch/Dir_Sense ==
  A : Inport
  B : Inport  Port=2
  Trigger : TriggerPort  VariantControl=Variant
  Constant : Constant  Value=-1
  Constant1 : Constant
  Logical Operator : Logic  AllPortsSameDT=off  OutDataTypeStr=boolean
  Switch : Switch  Criteria=u2 ~= 0  OutDataTypeStr=int16  SaturateOnIntegerOverflow=off  InputSameDT=off
  Sign : Outport  InitialOutput=0  VectorParamsAs1DForOutWhenUnconnected=off
  wires:
  Switch/1 -> Sign/1
  Constant1/1 -> Switch/3
  Constant/1 -> Switch/1
  Logical Operator/1 -> Switch/2
  B/1 -> Logical Operator/2
  A/1 -> Logical Operator/1

== system Design_of_an_Energy_Efficient_Hybrid_Electric_Vehicle/FOC/Speed Regulator1/Calculate position and speed/Sliding Mode Observer/Sliding Mode Observer/Direction_Latch/Subsystem2 ==
  SigmaAlpha : Inport
  SigmaBeta : Inport  Port=2
  Action Port : ActionPort
  Unary Minus : UnaryMinus
  Out1 : Outport
  Out2 : Outport  Port=2
  wires:
  Unary Minus/1 -> Out1/1
  SigmaBeta/1 -> Out2/1
  SigmaAlpha/1 -> Unary Minus/1

== system Design_of_an_Energy_Efficient_Hybrid_Electric_Vehicle/FOC/Speed Regulator1/Calculate position and speed/Sliding Mode Observer/Sliding Mode Observer/Direction_Latch/Subsystem3 ==
  SigmaBeta : Inport
  SigmaAlpha : Inport  Port=2
  Action Port : ActionPort
  Unary Minus : UnaryMinus
  Out2 : Outport
  Out1 : Outport  Port=2
  wires:
  Unary Minus/1 -> Out2/1
  SigmaAlpha/1 -> Out1/1
  SigmaBeta/1 -> Unary Minus/1

== system Design_of_an_Energy_Efficient_Hybrid_Electric_Vehicle/FOC/Speed Regulator1/Calculate position and speed/Sliding Mode Observer/Subsystem/Alpha_loop_current_est/Eq12_alpha_loop ==
  L*Zalpha[k+1] : Inport
  Valpha* : Inport  Port=2
  Reset : Inport  Port=3
  Add1 : Sum
  Add2 : Sum
  Delay1 : Delay  DelayLength=1  ExternalReset=Level
      settings: InputPortMap=u0,r5
  Delay2 : Delay  DelayLength=1  ExternalReset=Level
      settings: InputPortMap=u0,r5
  Gain : Gain  Gain=1/pmsm.Lq
  Gain1 : Gain  Gain=Ts
  Gain2 : Gain  Gain=(1-(Ts*pmsm.Rs/pmsm.Lq))
  Ialpha_est : Outport  VectorParamsAs1DForOutWhenUnconnected=off
  wires:
  Valpha*/1 -> Gain/1
  L*Zalpha[k+1]/1 -> Delay2/1
  Reset/1 -> Delay1/2, Delay2/2
  Delay2/1 -> Add1/1  "L*Zaplha[k]"
  Gain/1 -> Add1/2  "Valpha*/Lq"
  Add1/1 -> Gain1/1
  Delay1/1 -> Gain2/1
  Gain1/1 -> Add2/2
  Gain2/1 -> Add2/1
  Add2/1 -> Ialpha_est/1, Delay1/1  "Ialpha_est[k+1]"

== system Design_of_an_Energy_Efficient_Hybrid_Electric_Vehicle/FOC/Speed Regulator1/Calculate position and speed/Sliding Mode Observer/Subsystem/Beta_loop_current_est/Eq12_beta_loop ==
  L*Zbeta[k+1] : Inport
  Vbeta* : Inport  Port=2
  Reset : Inport  Port=3
  Add1 : Sum
  Add2 : Sum
  Delay1 : Delay  DelayLength=1  ExternalReset=Level
      settings: InputPortMap=u0,r5
  Delay2 : Delay  DelayLength=1  ExternalReset=Level
      settings: InputPortMap=u0,r5
  Gain : Gain  Gain=1/pmsm.Lq
  Gain1 : Gain  Gain=Ts
  Gain2 : Gain  Gain=(1-(Ts*pmsm.Rs/pmsm.Lq))
  Ibeta_est : Outport  VectorParamsAs1DForOutWhenUnconnected=off
  wires:
  Vbeta*/1 -> Gain/1
  L*Zbeta[k+1]/1 -> Delay2/1
  Reset/1 -> Delay1/2, Delay2/2
  Delay2/1 -> Add1/1  "L*Zbeta[k]"
  Gain/1 -> Add1/2  "Vbeta*/Lq"
  Add1/1 -> Gain1/1
  Delay1/1 -> Gain2/1
  Gain1/1 -> Add2/2
  Gain2/1 -> Add2/1
  Add2/1 -> Ibeta_est/1, Delay1/1  "Ibeta_est[k+1]"

== system Design_of_an_Energy_Efficient_Hybrid_Electric_Vehicle/FOC/Speed Regulator1/Calculate position and speed/Sliding Mode Observer/Subsystem/QPLL/Wrap state discrete Integrator ==
  u : Inport
  Add3 : Sum  Inputs=-+
  Constant3 : Constant  Value=2*pi
  Discrete-Time Integrator2 : DiscreteIntegrator  ExternalReset=rising  InitialConditionSource=external  SampleTime=-1  ShowStatePort=on  ICPrevOutput=DiscIntNeverNeededParam  ICPrevScaledInput=DiscIntNeverNeededParam
  Initial : InitialCondition  Value=0
  Relational Operator1 : RelationalOperator  Operator=>  OutDataTypeStr=boolean  InputSameDT=off
  Scope1 : Scope  NumInputPorts=2
  y : Outport  VectorParamsAs1DForOutWhenUnconnected=off
  wires:
  Discrete-Time Integrator2/1 -> Scope1/2, y/1
  u/1 -> Discrete-Time Integrator2/1
  Relational Operator1/1 -> Scope1/1, Discrete-Time Integrator2/2
  Initial/1 -> Discrete-Time Integrator2/3
  Constant3/1 -> Add3/1, Relational Operator1/2
  Add3/1 -> Initial/1
  Discrete-Time Integrator2/State -> Add3/2, Relational Operator1/1

== system Design_of_an_Energy_Efficient_Hybrid_Electric_Vehicle/FOC/Speed Regulator1/Calculate position and speed/Sliding Mode Observer/EEMF Model/Sliding Mode Observer/2nd order LPF/Compute filter constant ==
  Add : Sum  Inputs=+-
  Constant1 : Constant  Value=1 / (2*pi*fc)
  Constant2 : Constant
  Constant3 : Constant
  Divide : Product  Inputs=*/
  Weighted Sample Time1 : SampleTimeMath
  Weighted Sample Time2 : SampleTimeMath  TsampMathOp=Ts Only
  G : Outport
  wires:
  Constant3/1 -> Weighted Sample Time2/1
  Divide/1 -> Add/2  "α"
  Weighted Sample Time2/1 -> Divide/1
  Weighted Sample Time1/1 -> Divide/2
  Constant1/1 -> Weighted Sample Time1/1
  Constant2/1 -> Add/1
  Add/1 -> G/1

== system Design_of_an_Energy_Efficient_Hybrid_Electric_Vehicle/FOC/Speed Regulator1/Calculate position and speed/Sliding Mode Observer/EEMF Model/Sliding Mode Observer/2nd order LPF/LPF1 ==
  In : Inport
  rst : Inport  Port=2
  G : Inport  Port=3
  Add : Sum  Inputs=|++
  Constant : Constant  OutDataTypeStr=Inherit: Inherit via back propagation
  Data Type Conversion : DataTypeConversion  OutDataTypeStr=single  SaturateOnIntegerOverflow=off  RndMeth=Floor
  Delay : Delay  DelayLength=1  ExternalReset=Level hold
      settings: InputPortMap=u0,r5
  Minus : Sum  Inputs=+-
  Product : Product
  Product1 : Product
  Out : Outport
  wires:
  Minus/1 -> Product/2
  G/1 -> Minus/2, Product1/1
  Constant/1 -> Minus/1
  rst/1 -> Delay/2
  Delay/1 -> Product1/2
  In/1 -> Product/1
  Product/1 -> Add/1
  Product1/1 -> Add/2
  Add/1 -> Delay/1, Data Type Conversion/1
  Data Type Conversion/1 -> Out/1

== system Design_of_an_Energy_Efficient_Hybrid_Electric_Vehicle/FOC/Speed Regulator1/Calculate position and speed/Sliding Mode Observer/EEMF Model/Sliding Mode Observer/2nd order LPF/LPF2 ==
  In : Inport
  rst : Inport  Port=2
  G : Inport  Port=3
  Add : Sum  Inputs=|++
  Constant : Constant  OutDataTypeStr=Inherit: Inherit via back propagation
  Data Type Conversion : DataTypeConversion  OutDataTypeStr=single  SaturateOnIntegerOverflow=off  RndMeth=Floor
  Delay : Delay  DelayLength=1  ExternalReset=Level hold
      settings: InputPortMap=u0,r5
  Minus : Sum  Inputs=+-
  Product : Product
  Product1 : Product
  Out : Outport
  wires:
  Data Type Conversion/1 -> Out/1
  Add/1 -> Data Type Conversion/1, Delay/1
  Product1/1 -> Add/2
  Product/1 -> Add/1
  In/1 -> Product/1
  Delay/1 -> Product1/2
  rst/1 -> Delay/2
  Constant/1 -> Minus/1
  G/1 -> Product1/1, Minus/2
  Minus/1 -> Product/2

== system Design_of_an_Energy_Efficient_Hybrid_Electric_Vehicle/FOC/Speed Regulator1/Calculate position and speed/Sliding Mode Observer/EEMF Model/Sliding Mode Observer/Back EMF estimation (SMO)/Sigmoid ==
  u : Inport
  Demux : Demux  Outputs=2
  Mux : Mux  Inputs=2
  Sigmoid function : Fcn  Expr=(2/(1+exp(-a*u[1])))-1
  Sigmoid function1 : Fcn  Expr=(2/(1+exp(-a*u[1])))-1
  y : Outport
  wires:
  Demux/2 -> Sigmoid function1/1
  Demux/1 -> Sigmoid function/1
  u/1 -> Demux/1
  Sigmoid function1/1 -> Mux/2
  Sigmoid function/1 -> Mux/1
  Mux/1 -> y/1

== system Design_of_an_Energy_Efficient_Hybrid_Electric_Vehicle/FOC/Speed Regulator1/Calculate position and speed/Sliding Mode Observer/EEMF Model/Sliding Mode Observer/Speed//position estimation Arctan method/Rotor mechanical speed ==
  note: The rotor speed is obtained by differentiation of the measured angle. The function block removes angle discontinuities.
      |
      | The derivative is filtered to reduce the noise introduced by the numerical differentiation.
      |
      | See PN104: Using the angle decoder modules
      | on the imperix knowledge base (kb.imperix.com)
  angle : Inport
  reset : Inport  Port=2
  Angle derivator : Subsystem
  Low-pass filter : Subsystem
  speed : Outport
  wires:
  Low-pass filter/1(out) -> speed/1
  angle/1 -> Angle derivator/1(angle)
  reset/1 -> Low-pass filter/2(reset)
  Angle derivator/1(speed) -> Low-pass filter/1(in)

== system Design_of_an_Energy_Efficient_Hybrid_Electric_Vehicle/FOC/Speed Regulator1/Calculate position and speed/Sliding Mode Observer/EEMF Model/Sliding Mode Observer/Speed//position estimation Q-PLL method/PI ==
  e : Inport
  Kp : Inport  Port=2
  Ki : Inport  Port=3
  Reset : Inport  Port=4
  Add : Sum
  Discrete-Time Integrator : DiscreteIntegrator  ExternalReset=level  SampleTime=-1  OutDataTypeStr=single  ICPrevOutput=DiscIntNeverNeededParam  ICPrevScaledInput=DiscIntNeverNeededParam
  Product : Product
  Product1 : Product
  u : Outport
  wires:
  Kp/1 -> Product/1
  e/1 -> Product1/1, Product/2
  Product1/1 -> Discrete-Time Integrator/1
  Product/1 -> Add/1
  Discrete-Time Integrator/1 -> Add/2
  Ki/1 -> Product1/2
  Reset/1 -> Discrete-Time Integrator/2
  Add/1 -> u/1

== system Design_of_an_Energy_Efficient_Hybrid_Electric_Vehicle/FOC/Speed Regulator1/Calculate position and speed/Sliding Mode Observer/EEMF Model/Sliding Mode Observer/Speed//position estimation Q-PLL method/Wrapping integrator ==
  in : Inport
  Data Type Conversion : DataTypeConversion  OutDataTypeStr=single  SaturateOnIntegerOverflow=off  RndMeth=Floor
  Delay1 : Delay  DelayLength=1
  Delay2 : Delay  DelayLength=1
  Math Function : Math  Operator=mod  SignedPower=on  OutputSignalType=real
  Sample time : SampleTimeMath  TsampMathOp=*
  Sum1 : Sum  Inputs=|++  AccumDataTypeStr=single
  cst : Constant  Value=2*pi  OutDataTypeStr=Inherit: Inherit via back propagation  SampleTime=-1
  out : Outport
  wires:
  Delay2/1 -> out/1
  in/1 -> Sample time/1
  Math Function/1 -> Delay1/1, Delay2/1
  cst/1 -> Math Function/2
  Sample time/1 -> Data Type Conversion/1
  Sum1/1 -> Math Function/1
  Delay1/1 -> Sum1/2
  Data Type Conversion/1 -> Sum1/1

== system Design_of_an_Energy_Efficient_Hybrid_Electric_Vehicle/FOC/Speed Regulator1/Calculate position and speed/Sliding Mode Observer/EEMF Model/Sliding Mode Observer/Speed//position estimation Arctan method/Rotor mechanical speed/Angle derivator ==
  note: accounts for discontinuities in the measured angle
  angle : Inport
  Fcn : Fcn  Expr=u(1)+2*pi*((u(1)-u(2))<-pi)-2*pi*((u(1)-u(2)>pi))
  Mux : Mux  Inputs=2
  Sum : Sum  Inputs=|+-
  Unit Delay : UnitDelay  SampleTime=-1  HasFrameUpgradeWarning=on
  Weighted Sample Time : SampleTimeMath  TsampMathOp=/
  speed : Outport
  wires:
  Fcn/1 -> Sum/1
  Unit Delay/1 -> Mux/2, Sum/2
  Mux/1 -> Fcn/1
  angle/1 -> Unit Delay/1, Mux/1
  Weighted Sample Time/1 -> speed/1
  Sum/1 -> Weighted Sample Time/1

== system Design_of_an_Energy_Efficient_Hybrid_Electric_Vehicle/FOC/Speed Regulator1/Calculate position and speed/Sliding Mode Observer/EEMF Model/Sliding Mode Observer/Speed//position estimation Arctan method/Rotor mechanical speed/Low-pass filter ==
  note: fc = cut-off frequency (from mask)
      | Ts = sample time
      | tc = 1 / (2*pi*fc);
      | alpha = Ts / (tc + Ts);
  in : Inport
  reset : Inport  Port=2
  Compute alpha : Subsystem
  Constant : Constant  Value=fc  OutDataTypeStr=Inherit: Inherit via back propagation
  IIR : Subsystem  mask(Basic IIR LPF filter){}
      mask help:
      | The output is computed as:
      | y[k] = G * y[k-1] + (1-G) * u[k]
  out : Outport
  wires:
  in/1 -> IIR/2(u)
  reset/1 -> IIR/3(reset)
  IIR/1(y) -> out/1
  Constant/1 -> Compute alpha/1(fc)
  Compute alpha/1(α) -> IIR/1(α)

== system Design_of_an_Energy_Efficient_Hybrid_Electric_Vehicle/FOC/Speed Regulator1/Calculate position and speed/Sliding Mode Observer/EEMF Model/Sliding Mode Observer/Speed//position estimation Arctan method/Rotor mechanical speed/Low-pass filter/Compute alpha ==
  fc : Inport
  Fcn1 : Fcn  Expr=1/(2*pi*u(1))
  Fcn2 : Fcn  Expr=1/u(1)
  Weighted Sample Time1 : SampleTimeMath
  Weighted Sample Time2 : SampleTimeMath  TsampMathOp=*
  α : Outport
  wires:
  Fcn1/1 -> Weighted Sample Time1/1  "tc"
  fc/1 -> Fcn1/1
  Weighted Sample Time2/1 -> α/1  "Ts/(tc+Ts)"
  Fcn2/1 -> Weighted Sample Time2/1  "1/(tc+Ts)"
  Weighted Sample Time1/1 -> Fcn2/1  "tc+Ts"

== system Design_of_an_Energy_Efficient_Hybrid_Electric_Vehicle/FOC/Speed Regulator1/Calculate position and speed/Sliding Mode Observer/EEMF Model/Sliding Mode Observer/Speed//position estimation Arctan method/Rotor mechanical speed/Low-pass filter/IIR ==
  α : Inport
  u : Inport  Port=2
  reset : Inport  Port=3
  Add : Sum  Inputs=|++
  Constant : Constant  OutDataTypeStr=Inherit: Inherit via back propagation
  Data Type Conversion : DataTypeConversion  OutDataTypeStr=single  SaturateOnIntegerOverflow=off  RndMeth=Floor
  Delay : Delay  DelayLength=1  ExternalReset=Level hold
      settings: InputPortMap=u0,r5
  Product : Product
  Product1 : Product
  Subtract : Sum  Inputs=+-
  y : Outport
  wires:
  u/1 -> Product/1  "u[k]"
  Subtract/1 -> Product1/1  "(1-α)"
  α/1 -> Subtract/2, Product/2
  Constant/1 -> Subtract/1
  reset/1 -> Delay/2
  Delay/1 -> Product1/2  "y[k-1]"
  Product/1 -> Add/1  "α*u[k]"
  Product1/1 -> Add/2  "(1-α)*y[k-1]"
  Add/1 -> Data Type Conversion/1, Delay/1  "y[k] = (1-α) * y[k-1] + α * u[k]"
  Data Type Conversion/1 -> y/1

== matlab function Design_of_an_Energy_Efficient_Hybrid_Electric_Vehicle/FOC/Current reference calculation/MTPA Field Weakening Controller ==
  data: iqn_opt input; Ten input; iqn output; w input; Vdc input; params input; idn output
function [iqn,idn] = fcn(iqn_opt,Ten,w,Vdc,params)
% Maximum Torque Per Ampere (MTPA) Field Weakening Controller
% Olivier Tremblay, ETS 2008

kFact = 0.92; % safety factor 
Ld = params(1); % Ld inductance (H)
Lq = params(2); % Lq inductance (H)
lam = params(3); % Flux induced by magnets (Wb)
p = params(4); % Number of poles pairs
ib = params(5); % Base current
% Vs = Vdc/(pi/2)*kFact;  % Maximum operation with hysteresis modulation
Vs = Vdc/(sqrt(3))*kFact;  % Maximum operation with PWM 
ten = abs(Ten); %Normalized required torque
iqn = sign(Ten)*iqn_opt; %Normalized required q optimal current

if Ten == 0 && w == 0 % No speed and required torque = 0
    idn = 0;
elseif iqn ~= 0 % Normal operation, idn is a function of Ten and iqn
    idn = 1-Ten/iqn;
else %Special case if iqn = 0. To avoid zero division we calculate the current required to maintain speed
    idn = -(lam*p*w-Vs*kFact)/(p*Ld*w*ib);
end

%Overspeed: field weakening mode
if sqrt((-Lq*p*w*iqn*ib)^2+(Ld*p*w*idn*ib+lam*p*w)^2) >= Vs 
    vs = Vs;
    k1 = 2*lam*Ld/(ib*Lq^2);
    k2 = Ld^2/Lq^2;
    k3 = lam^2/(ib^2*Lq^2)+k2;
    
    g2 = -vs^2/(p^2*ib^2*Lq^2*w^2) + k1 + k3;
    g3 = -k1*ten-2*ten*k2;
    g4 = k2*ten^2;
    
    a1 = abs(-768*g4^3+384*g4^2*g2^2-48*g4*g2^4-432*g2*g4*g3^2+81*g3^4+12*g3^2*g2^3)^(1/2);
    a2 = (-288*g2*g4+108*g3^2+8*g2^3+12*a1)^(1/3);
    a3 = (-4*g2+a2+48/a2*g4+4/a2*g2^2)^(1/2);
    iqn = (1/12*6^(1/2)*a3+1/12*abs(-48*g2-6*a2-288/a2*g4-24/a2*g2^2-72/a3*g3*6^(1/2))^(1/2));
    iqn = sign(Ten)*iqn;

    idn = 1-Ten/iqn;
end

== matlab function Design_of_an_Energy_Efficient_Hybrid_Electric_Vehicle/SVPWM Modulator/MATLAB Function ==
  data: Ts parameter; Fsw parameter; Vref input; P output; PWMmethod parameter; D output; Clk input; Pavg parameter
function [P, D]   = ...
    UnifiedPWMModulator_2Levelx(Ts, Fsw, Vref, PWMmethod, Clk, Pavg)
[P, D]   = ...
    unifiedPWMModulator2Level(Ts, Fsw, Vref, PWMmethod, Pavg, Clk);
